simulink model "gryfModelBezPrzetwornikaIZaklucen"  (R2018b)
settings: Solver=VariableStepAuto  StartTime=0.0  StopTime=10  RelTol=1e-3
values from neighbouring files (symbols this model uses):
  Aw1 = pi*r1^2    (= 0.000804247719319)    [gryfBezPrzetwornikaIZaklucen.m]
  Aw2 = pi*r2^2    (= 0.000572555261117)    [gryfBezPrzetwornikaIZaklucen.m]
  g = 9.80665    [gryfBezPrzetwornikaIZaklucen.m]
  H1 = 1.9    [gryfBezPrzetwornikaIZaklucen.m]
  H10 = 0    [gryfBezPrzetwornikaIZaklucen.m]
  H2 = 1.55    [gryfBezPrzetwornikaIZaklucen.m]
  Hzad = 0.33    [gryfBezPrzetwornikaIZaklucen.m]
  R1 = D1/2    (= 0.45)    [gryfBezPrzetwornikaIZaklucen.m]
  R2 = D2/2    (= 0.35)    [gryfBezPrzetwornikaIZaklucen.m]
undefined symbols (not defined in the file or in its folder): h10
libraries: simulink x1
settings Model: Creator=gosci  LastModifiedBy=gosci

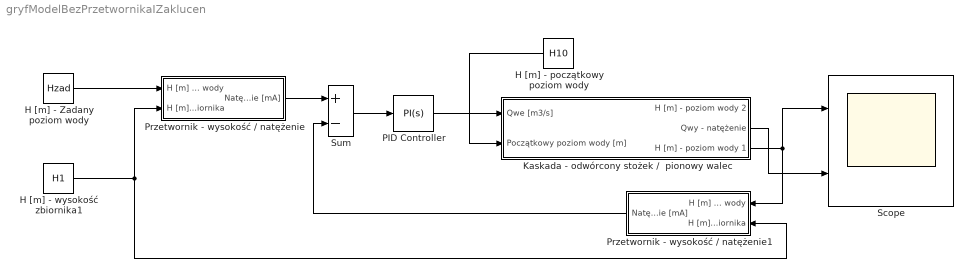
== system gryfModelBezPrzetwornikaIZaklucen ==
  H [m] - Zadany poziom wody : Constant  Value=Hzad
  H [m] - początkowy poziom wody : Constant  Value=H10
  H [m] - wysokość zbiornika1 : Constant  Value=H1
  Kaskada - odwórcony stożek /  pionowy walec : Subsystem
  PID Controller : simulink/Continuous/PID Controller  Controller=PI  Form=Parallel  TimeDomain=Continuous-time  SampleTime=-1  IntegratorMethod=Forward Euler  FilterMethod=Forward Euler  ControllerParametersSource=internal  P=13.8494634166043  I=92.0377495131412  D=-0.291455349658081  UseFilter=on  N=8.37231028830418  TunerSelectOption=Transfer Function Based (PID Tuner App)  InitialConditionSource=internal  InitialConditionForIntegrator=0  InitialConditionForFilter=0  DifferentiatorICPrevScaledInput=0  ExternalReset=none  TrackingMode=off  Kt=1  LimitOutput=off  UpperSaturationLimit=inf  LowerSaturationLimit=-inf  LinearizeAsGain=on  AntiWindupMode=none  Kb=1  POutMin=[]  POutMax=[]  IOutMin=[]  IOutMax=[]  DOutMin=[]  DOutMax=[]  NOutMin=[]  NOutMax=[]  SumOutMin=[]  SumOutMax=[]  SaturationOutMin=[]  SaturationOutMax=[]  PParamMin=[]  PParamMax=[]  IParamMin=[]  IParamMax=[]  DParamMin=[]  DParamMax=[]  NParamMin=[]  NParamMax=[]  KbParamMin=[]  KbParamMax=[]  KtParamMin=[]  KtParamMax=[]  KbOutMin=[]  KbOutMax=[]  KtOutMin=[]  KtOutMax=[]  IntegratorOutMin=[]  IntegratorOutMax=[]  FilterOutMin=[]  FilterOutMax=[]  SumI1OutMin=[]  SumI1OutMax=[]  SumI2OutMin=[]  SumI2OutMax=[]  SumI3OutMin=[]  SumI3OutMax=[]  SumI4OutMin=[]  SumI4OutMax=[]  SumDOutMin=[]  SumDOutMax=[]  DifferentiatorOutMin=[]  DifferentiatorOutMax=[]  FilterDiffOutCoefMin=[]  FilterDiffOutCoefMax=[]  ReciprocalOutMin=[]  ReciprocalOutMax=[]  SumDenOutMin=[]  SumDenOutMax=[]  SumNumOutMin=[]  SumNumOutMax=[]  DivideOutMin=[]  DivideOutMax=[]  IntegratorContinuousStateAttributes=''  IntegratorStateMustResolveToSignalObject=off  IntegratorRTWStateStorageClass=Auto  FilterContinuousStateAttributes=''  FilterStateMustResolveToSignalObject=off  FilterRTWStateStorageClass=Auto  ParallelPVariant=InternalParameters  IdealPVariant=Disabled  IVariant=InternalParameters  DVariant=Disabled  IntegratorVariant=Continuous  SatVariant=Disabled  AWVariant=Passthrough  PCopyVariant=Disabled  TRVariant=Disabled  FdbkBlocksVariant=Forward  IdealPFdbkVariant=Disabled  SatFdbkVariant=Disabled  DerivativeFilterVariant=Disabled  NVariant=Disabled  NCopyVariant=Disabled_SignalSpec  FilterICVariant=Disabled  IntegratorICVariant=InternalICs  ExternalResetVariant=Disabled  TRSumVariant=Passthrough  SumFdbkVariant=Disabled  SumVariant=Sum_PI
  Przetwornik - wysokość / natężenie : Subsystem
  Przetwornik - wysokość / natężenie1 : Subsystem
  Scope : Scope  NumInputPorts=2
  Sum : Sum  Inputs=+-
  wires:
  H [m] - początkowy poziom wody/1 -> Kaskada - odwórcony stożek /  pionowy walec/2(Początkowy poziom wody [m])
  Kaskada - odwórcony stożek /  pionowy walec/3(H [m] - poziom wody 1) -> Scope/1, Przetwornik - wysokość / natężenie1/1("H [m] - Poziom wody ")
  Kaskada - odwórcony stożek /  pionowy walec/2("Qwy - natężenie ") -> Scope/2
  Przetwornik - wysokość / natężenie1/1(Natężenie [mA]) -> Sum/2
  Przetwornik - wysokość / natężenie/1(Natężenie [mA]) -> Sum/1
  H [m] - Zadany poziom wody/1 -> Przetwornik - wysokość / natężenie/1("H [m] - Poziom wody ")
  H [m] - wysokość zbiornika1/1 -> Przetwornik - wysokość / natężenie1/2(H [m] - Wysokość zbiornika), Przetwornik - wysokość / natężenie/2(H [m] - Wysokość zbiornika)
  Sum/1 -> PID Controller/1
  PID Controller/1 -> Kaskada - odwórcony stożek /  pionowy walec/1("Qwe [m3/s] ")

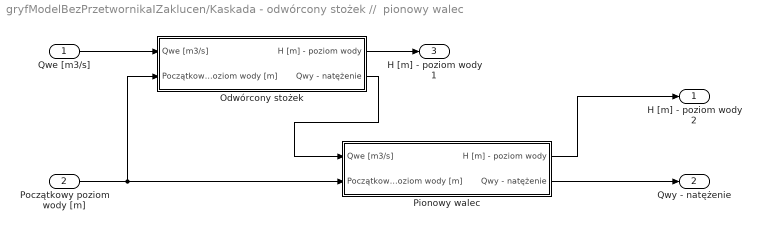
== system gryfModelBezPrzetwornikaIZaklucen/Kaskada - odwórcony stożek //  pionowy walec ==
  "Qwe [m3/s] " : Inport
  Początkowy poziom wody [m] : Inport  Port=2
  Odwórcony stożek : Subsystem
  Pionowy walec : Subsystem
  "H [m] - poziom wody 2 " : Outport
  "Qwy - natężenie " : Outport  Port=2
  H [m] - poziom wody 1 : Outport  Port=3
  wires:
  "Qwe [m3/s] "/1 -> Odwórcony stożek/1("Qwe [m3/s] ")
  Pionowy walec/1("H [m] - poziom wody ") -> "H [m] - poziom wody 2 "/1
  Pionowy walec/2("Qwy - natężenie ") -> "Qwy - natężenie "/1
  Początkowy poziom wody [m]/1 -> Odwórcony stożek/2(Początkowy poziom wody [m]), Pionowy walec/2(Początkowy poziom wody [m])
  Odwórcony stożek/1("H [m] - poziom wody ") -> H [m] - poziom wody 1/1
  Odwórcony stożek/2("Qwy - natężenie ") -> Pionowy walec/1("Qwe [m3/s] ")

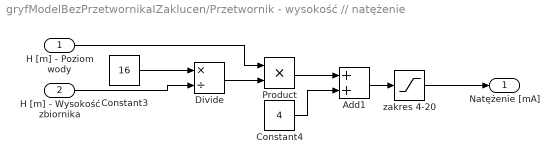
== system gryfModelBezPrzetwornikaIZaklucen/Przetwornik - wysokość // natężenie ==
  "H [m] - Poziom wody " : Inport
  H [m] - Wysokość zbiornika : Inport  Port=2
  Add1 : Sum
  Constant3 : Constant  Value=16
  Constant4 : Constant  Value=4
  Divide : Product  Inputs=*/
  Product : Product
  zakres 4-20 : Saturate  UpperLimit=20  LowerLimit=4
  Natężenie [mA] : Outport
  wires:
  Divide/1 -> Product/2
  zakres 4-20/1 -> Natężenie [mA]/1
  "H [m] - Poziom wody "/1 -> Product/1
  Add1/1 -> zakres 4-20/1
  Product/1 -> Add1/1
  H [m] - Wysokość zbiornika/1 -> Divide/2
  Constant3/1 -> Divide/1
  Constant4/1 -> Add1/2

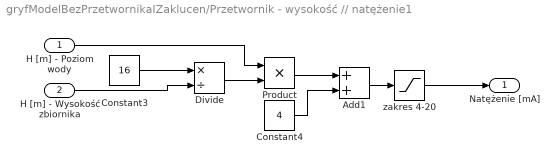
== system gryfModelBezPrzetwornikaIZaklucen/Przetwornik - wysokość // natężenie1 ==
  "H [m] - Poziom wody " : Inport
  H [m] - Wysokość zbiornika : Inport  Port=2
  Add1 : Sum
  Constant3 : Constant  Value=16
  Constant4 : Constant  Value=4
  Divide : Product  Inputs=*/
  Product : Product
  zakres 4-20 : Saturate  UpperLimit=20  LowerLimit=4
  Natężenie [mA] : Outport
  wires:
  Divide/1 -> Product/2
  zakres 4-20/1 -> Natężenie [mA]/1
  "H [m] - Poziom wody "/1 -> Product/1
  Add1/1 -> zakres 4-20/1
  Product/1 -> Add1/1
  H [m] - Wysokość zbiornika/1 -> Divide/2
  Constant3/1 -> Divide/1
  Constant4/1 -> Add1/2

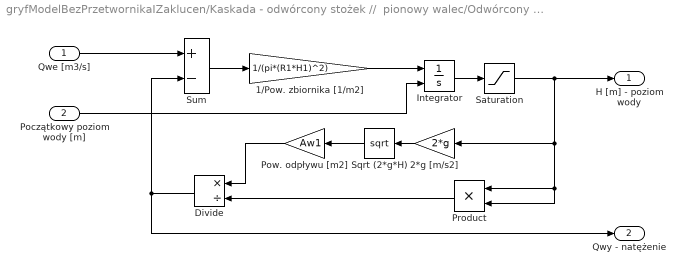
== system gryfModelBezPrzetwornikaIZaklucen/Kaskada - odwórcony stożek //  pionowy walec/Odwórcony stożek ==
  "Qwe [m3/s] " : Inport
  Początkowy poziom wody [m] : Inport  Port=2
  1/Pow. zbiornika [1/m2] : Gain  Gain=1/(pi*(R1*H1)^2)
  2*g [m/s2] : Gain  Gain=2*g
  Divide : Product  Inputs=*/
  Integrator : Integrator  InitialConditionSource=external  InitialCondition=h10
  Pow. odpływu [m2] : Gain  Gain=Aw1
  Product : Product
  Saturation : Saturate  UpperLimit=H1  LowerLimit=0.01
  Sqrt (2*g*H) : Sqrt  SaturateOnIntegerOverflow=on
  Sum : Sum  Inputs=+-
  "H [m] - poziom wody " : Outport
  "Qwy - natężenie " : Outport  Port=2
  wires:
  Sum/1 -> 1/Pow. zbiornika [1/m2]/1
  Saturation/1 -> 2*g [m/s2]/1, Product/1, Product/2, "H [m] - poziom wody "/1
  Sqrt (2*g*H)/1 -> Pow. odpływu [m2]/1
  "Qwe [m3/s] "/1 -> Sum/1
  1/Pow. zbiornika [1/m2]/1 -> Integrator/1
  2*g [m/s2]/1 -> Sqrt (2*g*H)/1
  Początkowy poziom wody [m]/1 -> Integrator/2
  Integrator/1 -> Saturation/1
  Product/1 -> Divide/2
  Pow. odpływu [m2]/1 -> Divide/1
  Divide/1 -> "Qwy - natężenie "/1, Sum/2

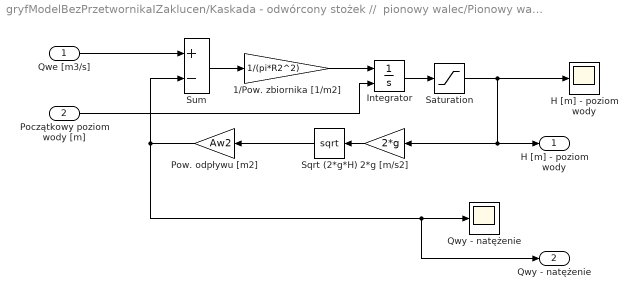
== system gryfModelBezPrzetwornikaIZaklucen/Kaskada - odwórcony stożek //  pionowy walec/Pionowy walec ==
  "Qwe [m3/s] " : Inport
  Początkowy poziom wody [m] : Inport  Port=2
  1/Pow. zbiornika [1/m2] : Gain  Gain=1/(pi*R2^2)
  2*g [m/s2] : Gain  Gain=2*g
  H [m] - poziom wody : Scope
  Integrator : Integrator  InitialConditionSource=external  InitialCondition=h10
  Pow. odpływu [m2] : Gain  Gain=Aw2
  Qwy - natężenie : Scope
  Saturation : Saturate  UpperLimit=H2  LowerLimit=0.01
  Sqrt (2*g*H) : Sqrt  SaturateOnIntegerOverflow=on
  Sum : Sum  Inputs=+-
  "H [m] - poziom wody " : Outport
  "Qwy - natężenie " : Outport  Port=2
  wires:
  Sum/1 -> 1/Pow. zbiornika [1/m2]/1
  Saturation/1 -> H [m] - poziom wody/1, 2*g [m/s2]/1, "H [m] - poziom wody "/1
  Pow. odpływu [m2]/1 -> "Qwy - natężenie "/1, Qwy - natężenie/1, Sum/2
  Sqrt (2*g*H)/1 -> Pow. odpływu [m2]/1
  "Qwe [m3/s] "/1 -> Sum/1
  1/Pow. zbiornika [1/m2]/1 -> Integrator/1
  2*g [m/s2]/1 -> Sqrt (2*g*H)/1
  Początkowy poziom wody [m]/1 -> Integrator/2
  Integrator/1 -> Saturation/1
